simulink model "Zad2"  (R2020b)
settings: Solver=VariableStepAuto  StartTime=0.0  StopTime=0.0  RelTol=1e-3
libraries: CPOiS_SourcesSinks x5, CPOiS_LinearTransforms x2, CPOiS_DataManipulation_DataTypeConversion x2, CPOiS_Edges x1, CPOiS_General x1
settings Model: Creator=Krystian  LastModifiedBy=Krystian

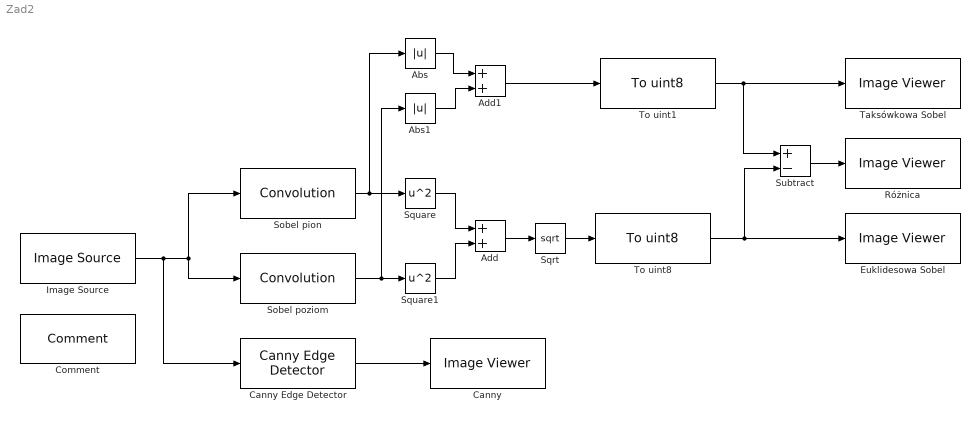
== system Zad2 ==
  Abs : Abs
  Abs1 : Abs
  Add : Sum
  Add1 : Sum
  "Canny " : CPOiS_SourcesSinks/Image Viewer
      settings: SourceProductName=CPOiS - Digital image and signal processing
  Canny Edge Detector : CPOiS_Edges/Canny Edge Detector  LowThresh=50  HighThresh=100
      settings: SourceProductName=CPOiS - Digital image and signal processing
  Comment : CPOiS_General/Comment
      settings: SourceProductName=CPOiS - Digital image and signal processing
  Euklidesowa Sobel : CPOiS_SourcesSinks/Image Viewer
      settings: SourceProductName=CPOiS - Digital image and signal processing
  Image Source : CPOiS_SourcesSinks/Image Source  FileSelection=cameraman.tif
      settings: SourceProductName=CPOiS - Digital image and signal processing
  Różnica : CPOiS_SourcesSinks/Image Viewer
      settings: SourceProductName=CPOiS - Digital image and signal processing
  Sobel pion : CPOiS_LinearTransforms/Convolution  ConvolutionMatrix=[-1,0,1;-2,0,2;-1,0,1]
      settings: SourceProductName=CPOiS - Digital image and signal processing
  Sobel poziom : CPOiS_LinearTransforms/Convolution  ConvolutionMatrix=[-1,-2,-1;0,0,0;1,2,1]
      settings: SourceProductName=CPOiS - Digital image and signal processing
  Sqrt : Sqrt  SaturateOnIntegerOverflow=on
  Square : Math  Operator=square  SignedPower=on  SaturateOnIntegerOverflow=on
  Square1 : Math  Operator=square  SignedPower=on  SaturateOnIntegerOverflow=on
  Subtract : Sum  Inputs=+-
  Taksówkowa Sobel : CPOiS_SourcesSinks/Image Viewer
      settings: SourceProductName=CPOiS - Digital image and signal processing
  To uint1 : CPOiS_DataManipulation_DataTypeConversion/To uint8
      settings: SourceProductName=CPOiS - Digital image and signal processing
  To uint8 : CPOiS_DataManipulation_DataTypeConversion/To uint8
      settings: SourceProductName=CPOiS - Digital image and signal processing
  wires:
  Add1/1 -> To uint1/1
  Square/1 -> Add/1
  Square1/1 -> Add/2
  To uint8/1 -> Euklidesowa Sobel/1, Subtract/2
  Sqrt/1 -> To uint8/1
  Sobel pion/1 -> Abs/1, Square/1
  Image Source/1 -> Canny Edge Detector/1, Sobel pion/1, Sobel poziom/1
  Sobel poziom/1 -> Square1/1, Abs1/1
  Abs1/1 -> Add1/2
  Abs/1 -> Add1/1
  Canny Edge Detector/1 -> "Canny "/1
  To uint1/1 -> Subtract/1, Taksówkowa Sobel/1
  Add/1 -> Sqrt/1
  Subtract/1 -> Różnica/1
